simulink model "WF_offshore"  (R2024a)
settings: Solver=VariableStepAuto  StartTime=0  StopTime=1  RelTol=1e-3
values from neighbouring files (symbols this model uses):
  c_c = 0.177e-6    (= 1.77e-07)    [WF_onshore_SSO_GFL.m]    (also in WF_physical_param_offshore_supersynchronous.m = cable_220(i,6)*1e-9; WF_physical_param_onshore_SSO_020625.m = cable_220(i,6)*1e-9; initialize_params_agg.m)
  c_c_eff = c_c*n_cables    [WF_onshore_SSO_GFL.m]    (also in WF_physical_param_offshore_supersynchronous.m; WF_physical_param_onshore_SSO_020625.m; initialize_params_agg.m)
  cvtr = initialize_NR_VSC_GF(cvtr)    [NR_steadystate_VSC_GF.m]    (also in WF_onshore_SSO_GFL.m = setfield(cvtr,'parameters', p_vary.name,p_vary.val(i)); WF_physical_param_offshore_supersynchronous.m = setfield(cvtr,'parameters', p_vary.name,p_vary.val(i)); WF_physical_param_onshore_SSO_020625.m = setfield(cvtr,'parameters', p_vary.name,p_vary.val(i)); impedance_WT_blackbox.m = base_values(cvtr))
  D_C = 10:4:100    [WF_onshore_SSO_GFL.m]    (also in WF_parameter_variation.m = 10:4:150; WF_physical_param.m = 10:4:150; WF_physical_param_offshore_supersynchronous.m = 50; WF_physical_param_onshore_SSO_020625.m = 50)
  enable_pll = 1    [impedance_WT_agg.m]    (also in initialize_WT_agg.m; initialize_WT_default_gfl.m; initialize_WT_default_offshore_super.m)
  f1 = 50    [WF_onshore_SSO_GFL.m]    (also in WF_physical_param_offshore_supersynchronous.m; WF_physical_param_onshore_SSO_020625.m; initialize_params_agg.m)
  i = 1    [WF_physical_param_offshore_supersynchronous.m]    (also in WF_physical_param_onshore_SSO_020625.m)
  L = inv(R)    [participation_factors_VSC_GF.m]
  l_c = 0.386e-3    (= 0.000386)    [WF_onshore_SSO_GFL.m]    (also in WF_physical_param_offshore_supersynchronous.m = cable_220(i,5)*1e-3; WF_physical_param_onshore_SSO_020625.m = cable_220(i,5)*1e-3; initialize_params_agg.m)
  l_c_eff = l_c/n_cables    [WF_onshore_SSO_GFL.m]    (also in WF_physical_param_offshore_supersynchronous.m; WF_physical_param_onshore_SSO_020625.m; initialize_params_agg.m)
  L_comp = sqrt(2)*l_comp*(Z_b_G/(2*pi*f1))    [WF_physical_param.m]    (also in WF_physical_param_offshore_supersynchronous.m = sqrt(2)*((1/(c_c_eff/2*D_C*2*pi*f1))-(l_tf_wf*(Z_b_G)+(l_c_e; WF_physical_param_onshore_SSO_020625.m = sqrt(2)*((1/(c_c_eff/2*D_C*2*pi*f1))-(l_tf_wf*(Z_b_G)+(l_c_e; initialize_params_agg.m)
  l_OH = 0.2    [WF_onshore_SSO_GFL.m]    (also in WF_physical_param_offshore_supersynchronous.m = 0.1; WF_physical_param_onshore_SSO_020625.m = 0.1; initialize_params_agg.m = 0.1)
  l_tf_wf = tf_params(2,2)    [IM_WF_agg.m]    (also in WF_onshore_SSO_GFL.m = 0.05; WF_physical_param_offshore_supersynchronous.m = 0.05; WF_physical_param_onshore_SSO_020625.m = 0.05; initialize_params_agg.m = 0.05)
  l_tf_wt = tf_params(1,2)    [IM_WF_agg.m]    (also in WF_onshore_SSO_GFL.m = 0.0392; WF_physical_param_offshore_supersynchronous.m = 0.0392; WF_physical_param_onshore_SSO_020625.m = 0.0392; initialize_params_agg.m = 0.0392)
  Lg = p_vary(i)*((Z_b_G/(2*pi*f1)))    [WF_onshore_SSO_GFL.m]    (also in WF_physical_param_offshore_supersynchronous.m; WF_physical_param_onshore_SSO_020625.m; initialize_params_agg.m = 0.1*((Z_b_G/(2*pi*f1))))
  Lg1 = Lg    [WF_physical_param_offshore_supersynchronous.m]    (also in WF_physical_param_onshore_SSO_020625.m)
  Lg2 = Lg    [WF_physical_param_offshore_supersynchronous.m]    (also in WF_physical_param_onshore_SSO_020625.m)
  r_c = 27e-3    (= 0.027)    [WF_onshore_SSO_GFL.m]    (also in WF_physical_param_offshore_supersynchronous.m = cable_220(i,4)*1e-3; WF_physical_param_onshore_SSO_020625.m = cable_220(i,4)*1e-3; initialize_params_agg.m)
  r_c_eff = r_c/n_cables    [WF_onshore_SSO_GFL.m]    (also in WF_physical_param_offshore_supersynchronous.m; WF_physical_param_onshore_SSO_020625.m; initialize_params_agg.m)
  r_diss = .1    (= 0.1)    [WF_physical_param_offshore_supersynchronous.m]    (also in WF_physical_param_onshore_SSO_020625.m; calculate_WF.m; initialize_params_agg.m)
  r_OH = 0.02    [WF_onshore_SSO_GFL.m]    (also in WF_physical_param_offshore_supersynchronous.m = 0.01; WF_physical_param_onshore_SSO_020625.m = 0.01; initialize_params_agg.m)
  r_tf_wf = tf_params(2,1)    [IM_WF_agg.m]    (also in WF_onshore_SSO_GFL.m = 0.005; WF_physical_param_offshore_supersynchronous.m = 0.005; WF_physical_param_onshore_SSO_020625.m = 0.005; initialize_params_agg.m = 0.005)
  r_tf_wt = tf_params(1,1)    [IM_WF_agg.m]    (also in WF_onshore_SSO_GFL.m = 0.0056; WF_physical_param_offshore_supersynchronous.m = 0.0056; WF_physical_param_onshore_SSO_020625.m = 0.0056; initialize_params_agg.m = 0.0056)
  Rg = rg*Z_b_G    [WF_onshore_SSO_GFL.m]    (also in WF_physical_param_offshore_supersynchronous.m; WF_physical_param_onshore_SSO_020625.m; initialize_params_agg.m = 0.01*Z_b_G)
  Sb_WF = (3*1)*5e6    (= 15000000)    [WF_onshore_SSO_GFL.m]    (also in WF_physical_param_offshore_supersynchronous.m; WF_physical_param_onshore_SSO_020625.m; impedance_WT_blackbox.m = n_t*Sb_WT; initialize_params_agg.m = 1000000000)
  Sb_WT = 5e6    (= 5000000)    [IM_WF.m]    (also in WF_onshore_SSO_GFL.m; WF_physical_param_offshore_supersynchronous.m; WF_physical_param_onshore_SSO_020625.m; initialize_params_agg.m)
  selector_current_reference = 3    [impedance_WT_agg.m]    (also in initialize_WT_agg.m; initialize_WT_default_gfl.m; initialize_WT_default_offshore_super.m)
  selector_omega_reference = 1    [impedance_WT_agg.m]    (also in initialize_WT_agg.m; initialize_WT_default_gfl.m; initialize_WT_default_offshore_super.m)
  V_coll = 33e3    (= 33000)    [WF_onshore_SSO_GFL.m]    (also in WF_physical_param_offshore_supersynchronous.m; WF_physical_param_onshore_SSO_020625.m; initialize_params_agg.m)
  V_trans = 220e3    (= 220000)    [WF_onshore_SSO_GFL.m]    (also in WF_physical_param_offshore_supersynchronous.m; WF_physical_param_onshore_SSO_020625.m; initialize_params_agg.m)
  Z_b_G = (V_trans/sqrt(3/2))^2/Sb_WF    [WF_onshore_SSO_GFL.m]    (also in WF_physical_param_offshore_supersynchronous.m = (V_b_trans)^2/Sb_WF; WF_physical_param_onshore_SSO_020625.m = (V_b_trans)^2/Sb_WF; initialize_params_agg.m = (V_b_trans)^2/Sb_WF)
undefined symbols (not defined in the file or in its folder): opts, R
libraries: spsSeriesRLCBranchLib x105, simulink_extras x104, simulink x52, spsThreePhaseVIMeasurementLib x42, spsControlledVoltageSourceLib x42, spsGroundLib x41, spsThreePhaseTransformerTwoWindingsLib x14, powerlib_extras x13, spsVariableInductorLib x9, spsIdealSwitchLib x6, spsVariableCapacitorLib x6, spsThreePhaseSeriesRLCBranchLib x4
(part 2 of 13)

== system WF_offshore/WT_MF14 ==
  Control System : Subsystem  mask{Ts_control=cvtr.parameters.T_cont}
      mask prompts: Ts_control "Sample Time"
  Gain1 : Gain  Gain=1/cvtr.pu.Vb
  Gain2 : Gain  Gain=1/cvtr.pu.Ib
  Gain5 : Gain  Gain=cvtr.pu.Vb
  I_conv : ToWorkspace  VariableName=I_conv  SaveFormat=Structure With Time  SampleTime=-1
      settings: MaxDataPoints=1000000
  Inverse Park1 : Subsystem
  Scope2 : Scope  NumInputPorts=2
  Subsystem1 : Subsystem
  Subsystem6 : Subsystem
  Three-Phase Transformer (Two Windings) : spsThreePhaseTransformerTwoWindingsLib/Three-Phase Transformer (Two Windings)  Winding1Connection=Yg  Winding2Connection=Yg  CoreType=Three single-phase transformers  SetSaturation=off  Hysteresis=off  DataFile='hysteresis'  SetInitialFlux=off  Measurements=None  UNITS=pu  NominalPower=[Sb_WF , f1 ]  Winding1=[ cvtr.parameters.Vnr ,r_tf_wt/2 , l_tf_wt/2]  Winding2=[ V_coll , r_tf_wt/2, l_tf_wt/2]  Rm=5000  Lm=0  L0=0.5  Saturation=[ 0,0 ; 0.0024,1.2 ; 1.0,1.52 ]  InitialFluxes=[ 0.8 , -0.8 , 0.7 ]  BreakLoop=off  DiscreteSolver=Trapezoidal iterative  DataType=off  TransfoNumber=1
  Three-Phase V-I Measurement : spsThreePhaseVIMeasurementLib/Three-Phase V-I Measurement  VoltageMeasurement=phase-to-ground  SetLabelV=off  LabelV=Vabc  Vpu=off  VpuLL=off  CurrentMeasurement=yes  SetLabelI=off  LabelI=Iabc  Ipu=off  Pbase=100e6  Vbase=500e3  OutputType=Complex  PhasorSimulation=off  PSBequivalent=0
  Transformations (pu and dq) : Subsystem
  V_conv : ToWorkspace  VariableName=V_conv  SaveFormat=Structure With Time  SampleTime=-1
      settings: MaxDataPoints=1000000
  filter capacitance1 : Subsystem
      settings: PortSchema="{\"entries\":[{\"content\":{\"sides\":[{\"content\":{\"connectorIds\":[\"LConn1\",\"LConn2\",\"LConn3\"]},\"type\":\"ConnectorPlacement.EquallySpacedRectSide\",\"uuid\":\"e81be3d5-6303-4565-8ca3-afc618f21d70\"},{\"content\":{\"connectorIds\":[],\"side\":\"RIGHT\"},\"type\":\"ConnectorPlacement.EquallySpacedRectSide\",\"uuid\":\"458d9030-e614-487d-87de-3e53be7c7da4\"},{\"content\":{\"connectorIds\":[],\"side\":\"TOP\"},\"type\":\"ConnectorPlacement.EquallySpacedRectSide\",\"uuid\":\"a29d66a0-f095-498d-bb9b-96c7f47699d3\"},{\"content\":{\"connectorIds\":[\"Out1\"],\"side\":\"BOTTOM\"},\"type\":\"ConnectorPlacement.EquallySpacedRectSide\",\"uuid\":\"afc68874-c098-43f5-9b37-53a3b484513b\"}]},\"type\":\"ConnectorPlacement.EquallySpacedConnector\",\"uuid\":\"37f495dd-1c12-4bb8-af72-7ef46bbd951c\"}],\"packageUris\":[\"http://schema.mathworks.com/mf0/Connector/R2020b\"],\"version\":\"1.0\"}"
  filter inductance1 : Subsystem
      settings: PortSchema="{\"entries\":[{\"content\":{\"sides\":[{\"content\":{\"connectorIds\":[\"LConn1\",\"LConn2\",\"LConn3\"]},\"type\":\"ConnectorPlacement.EquallySpacedRectSide\",\"uuid\":\"d3d60048-9578-4fa3-8d11-9c8a66a4b1f9\"},{\"content\":{\"connectorIds\":[\"RConn1\",\"RConn2\",\"RConn3\"],\"side\":\"RIGHT\"},\"type\":\"ConnectorPlacement.EquallySpacedRectSide\",\"uuid\":\"184a2c1d-36ab-46d1-99e4-db01aa31ec94\"},{\"content\":{\"connectorIds\":[\"Out1\"],\"side\":\"TOP\"},\"type\":\"ConnectorPlacement.EquallySpacedRectSide\",\"uuid\":\"db651021-9d7f-4124-8d21-ede853163467\"}]},\"type\":\"ConnectorPlacement.EquallySpacedConnector\",\"uuid\":\"723d0964-19fd-4dbe-91e3-e4ea0bb1cca9\"}],\"packageUris\":[\"http://schema.mathworks.com/mf0/Connector/R2020b\"],\"version\":\"1.0\"}"
  a : PMIOPort  Side=Right
  b : PMIOPort  Port=2  Side=Right
  c : PMIOPort  Port=3  Side=Right
  wires:
  Control System/2(thetavsm) -> [Thetavsm]
  Control System/3(vir) -> [vir]
  Control System/1(thetapll) -> [Thetapll]
  Transformations (pu and dq)/2(il) -> Control System/2(il)  "il"
  Transformations (pu and dq)/1(io) -> Control System/1(io)  "io"
  Transformations (pu and dq)/3(p) -> Control System/3(p)  "p"
  Transformations (pu and dq)/4(q) -> Control System/4(q)  "q"
  Transformations (pu and dq)/5(vo_pll) -> Control System/5(vo_pll)  "vo_pll"
  Transformations (pu and dq)/6(vo) -> Control System/6(vo)  "vo"
  [Thetavsm] -> Transformations (pu and dq)/5(Thetavsm)
  [Thetapll] -> Transformations (pu and dq)/6(Thetapll)
  [vir] -> Gain5/1
  Subsystem6/1(x_dq) -> Inverse Park1/1(x_dq)
  Gain5/1 -> Subsystem6/1(x_d+ix_q)
  Three-Phase V-I Measurement/2 -> Gain2/1, [i_abc_grid]  "i_abc_grid"
  Inverse Park1/1(x_abc) -> Subsystem1/1(v_abc)
  Three-Phase V-I Measurement/1 -> Gain1/1, [v_abc_grid]  "v_abc_grid"
  [Thetavsm] -> Inverse Park1/2(delta)
  filter capacitance1/1(v_abc) -> [v_abc_filt]  "v_abc_filt"
  filter inductance1/1(i_abc) -> [i_abc_filt]  "i_abc_filt"
  [v_abc_grid] -> Transformations (pu and dq)/3(v_abc_grid)
  [v_abc_filt] -> Transformations (pu and dq)/4(v_abc_filt)
  [i_abc_filt] -> Transformations (pu and dq)/2(i_abc_filt)
  [i_abc_grid] -> Transformations (pu and dq)/1(i_abc_grid)
  Gain1/1 -> Scope2/1, V_conv/1
  Gain2/1 -> Scope2/2, I_conv/1
  connections:
  filter inductance1/RConn3 -- filter capacitance1/LConn3 -- Three-Phase V-I Measurement/LConn3
  filter inductance1/RConn1 -- filter capacitance1/LConn1 -- Three-Phase V-I Measurement/LConn1
  filter inductance1/RConn2 -- filter capacitance1/LConn2 -- Three-Phase V-I Measurement/LConn2
  Subsystem1/RConn1 -- filter inductance1/LConn1
  Subsystem1/RConn2 -- filter inductance1/LConn2
  Subsystem1/RConn3 -- filter inductance1/LConn3
  Three-Phase Transformer (Two Windings)/RConn1 -- a/RConn1
  Three-Phase Transformer (Two Windings)/RConn2 -- b/RConn1
  Three-Phase Transformer (Two Windings)/RConn3 -- c/RConn1
  Three-Phase Transformer (Two Windings)/LConn1 -- Three-Phase V-I Measurement/RConn1
  Three-Phase Transformer (Two Windings)/LConn2 -- Three-Phase V-I Measurement/RConn2
  Three-Phase Transformer (Two Windings)/LConn3 -- Three-Phase V-I Measurement/RConn3

== system WF_offshore/WT_MF2 ==
  Control System : Subsystem  mask{Ts_control=cvtr.parameters.T_cont}
      mask prompts: Ts_control "Sample Time"
  Gain5 : Gain  Gain=cvtr.pu.Vb
  Inverse Park1 : Subsystem
  Subsystem1 : Subsystem
  Subsystem6 : Subsystem
  Three-Phase Transformer (Two Windings) : spsThreePhaseTransformerTwoWindingsLib/Three-Phase Transformer (Two Windings)  Winding1Connection=Yg  Winding2Connection=Yg  CoreType=Three single-phase transformers  SetSaturation=off  Hysteresis=off  DataFile='hysteresis'  SetInitialFlux=off  Measurements=None  UNITS=pu  NominalPower=[Sb_WT, f1 ]  Winding1=[ cvtr.parameters.Vnr ,r_tf_wt/2 , l_tf_wt/2]  Winding2=[ V_coll , r_tf_wt/2, l_tf_wt/2]  Rm=5000  Lm=0  L0=0.5  Saturation=[ 0,0 ; 0.0024,1.2 ; 1.0,1.52 ]  InitialFluxes=[ 0.8 , -0.8 , 0.7 ]  BreakLoop=off  DiscreteSolver=Trapezoidal iterative  DataType=off  TransfoNumber=1
  Three-Phase V-I Measurement : spsThreePhaseVIMeasurementLib/Three-Phase V-I Measurement  VoltageMeasurement=phase-to-ground  SetLabelV=off  LabelV=Vabc  Vpu=off  VpuLL=off  CurrentMeasurement=yes  SetLabelI=off  LabelI=Iabc  Ipu=off  Pbase=100e6  Vbase=500e3  OutputType=Complex  PhasorSimulation=off  PSBequivalent=0
  Transformations (pu and dq) : Subsystem
  filter capacitance1 : Subsystem
      settings: PortSchema="{\"entries\":[{\"content\":{\"sides\":[{\"content\":{\"connectorIds\":[\"LConn1\",\"LConn2\",\"LConn3\"]},\"type\":\"ConnectorPlacement.EquallySpacedRectSide\",\"uuid\":\"e81be3d5-6303-4565-8ca3-afc618f21d70\"},{\"content\":{\"connectorIds\":[],\"side\":\"RIGHT\"},\"type\":\"ConnectorPlacement.EquallySpacedRectSide\",\"uuid\":\"458d9030-e614-487d-87de-3e53be7c7da4\"},{\"content\":{\"connectorIds\":[],\"side\":\"TOP\"},\"type\":\"ConnectorPlacement.EquallySpacedRectSide\",\"uuid\":\"a29d66a0-f095-498d-bb9b-96c7f47699d3\"},{\"content\":{\"connectorIds\":[\"Out1\"],\"side\":\"BOTTOM\"},\"type\":\"ConnectorPlacement.EquallySpacedRectSide\",\"uuid\":\"afc68874-c098-43f5-9b37-53a3b484513b\"}]},\"type\":\"ConnectorPlacement.EquallySpacedConnector\",\"uuid\":\"37f495dd-1c12-4bb8-af72-7ef46bbd951c\"}],\"packageUris\":[\"http://schema.mathworks.com/mf0/Connector/R2020b\"],\"version\":\"1.0\"}"
  filter inductance1 : Subsystem
      settings: PortSchema="{\"entries\":[{\"content\":{\"sides\":[{\"content\":{\"connectorIds\":[\"LConn1\",\"LConn2\",\"LConn3\"]},\"type\":\"ConnectorPlacement.EquallySpacedRectSide\",\"uuid\":\"d3d60048-9578-4fa3-8d11-9c8a66a4b1f9\"},{\"content\":{\"connectorIds\":[\"RConn1\",\"RConn2\",\"RConn3\"],\"side\":\"RIGHT\"},\"type\":\"ConnectorPlacement.EquallySpacedRectSide\",\"uuid\":\"184a2c1d-36ab-46d1-99e4-db01aa31ec94\"},{\"content\":{\"connectorIds\":[\"Out1\"],\"side\":\"TOP\"},\"type\":\"ConnectorPlacement.EquallySpacedRectSide\",\"uuid\":\"db651021-9d7f-4124-8d21-ede853163467\"}]},\"type\":\"ConnectorPlacement.EquallySpacedConnector\",\"uuid\":\"723d0964-19fd-4dbe-91e3-e4ea0bb1cca9\"}],\"packageUris\":[\"http://schema.mathworks.com/mf0/Connector/R2020b\"],\"version\":\"1.0\"}"
  a : PMIOPort  Side=Right
  b : PMIOPort  Port=2  Side=Right
  c : PMIOPort  Port=3  Side=Right
  wires:
  [i_abc_grid] -> Transformations (pu and dq)/1(i_abc_grid)
  [i_abc_filt] -> Transformations (pu and dq)/2(i_abc_filt)
  [v_abc_filt] -> Transformations (pu and dq)/4(v_abc_filt)
  [v_abc_grid] -> Transformations (pu and dq)/3(v_abc_grid)
  filter inductance1/1(i_abc) -> [i_abc_filt]  "i_abc_filt"
  filter capacitance1/1(v_abc) -> [v_abc_filt]  "v_abc_filt"
  [Thetavsm] -> Inverse Park1/2(delta)
  Three-Phase V-I Measurement/1 -> [v_abc_grid]  "v_abc_grid"
  Inverse Park1/1(x_abc) -> Subsystem1/1(v_abc)
  Three-Phase V-I Measurement/2 -> [i_abc_grid]  "i_abc_grid"
  Gain5/1 -> Subsystem6/1(x_d+ix_q)
  Subsystem6/1(x_dq) -> Inverse Park1/1(x_dq)
  [vir] -> Gain5/1
  [Thetapll] -> Transformations (pu and dq)/6(Thetapll)
  [Thetavsm] -> Transformations (pu and dq)/5(Thetavsm)
  Transformations (pu and dq)/6(vo) -> Control System/6(vo)  "vo"
  Transformations (pu and dq)/5(vo_pll) -> Control System/5(vo_pll)  "vo_pll"
  Transformations (pu and dq)/4(q) -> Control System/4(q)  "q"
  Transformations (pu and dq)/3(p) -> Control System/3(p)  "p"
  Transformations (pu and dq)/1(io) -> Control System/1(io)  "io"
  Transformations (pu and dq)/2(il) -> Control System/2(il)  "il"
  Control System/1(thetapll) -> [Thetapll]
  Control System/3(vir) -> [vir]
  Control System/2(thetavsm) -> [Thetavsm]
  connections:
  Three-Phase Transformer (Two Windings)/LConn3 -- Three-Phase V-I Measurement/RConn3
  Three-Phase Transformer (Two Windings)/LConn2 -- Three-Phase V-I Measurement/RConn2
  Three-Phase Transformer (Two Windings)/LConn1 -- Three-Phase V-I Measurement/RConn1
  Three-Phase Transformer (Two Windings)/RConn3 -- c/RConn1
  Three-Phase Transformer (Two Windings)/RConn2 -- b/RConn1
  Three-Phase Transformer (Two Windings)/RConn1 -- a/RConn1
  Subsystem1/RConn3 -- filter inductance1/LConn3
  Subsystem1/RConn2 -- filter inductance1/LConn2
  Subsystem1/RConn1 -- filter inductance1/LConn1
  Three-Phase V-I Measurement/LConn2 -- filter capacitance1/LConn2 -- filter inductance1/RConn2
  Three-Phase V-I Measurement/LConn1 -- filter capacitance1/LConn1 -- filter inductance1/RConn1
  Three-Phase V-I Measurement/LConn3 -- filter capacitance1/LConn3 -- filter inductance1/RConn3

== system WF_offshore/WT_MF3 ==
  Control System : Subsystem  mask{Ts_control=cvtr.parameters.T_cont}
      mask prompts: Ts_control "Sample Time"
  Gain5 : Gain  Gain=cvtr.pu.Vb
  Inverse Park1 : Subsystem
  Subsystem1 : Subsystem
  Subsystem6 : Subsystem
  Three-Phase Transformer (Two Windings) : spsThreePhaseTransformerTwoWindingsLib/Three-Phase Transformer (Two Windings)  Winding1Connection=Yg  Winding2Connection=Yg  CoreType=Three single-phase transformers  SetSaturation=off  Hysteresis=off  DataFile='hysteresis'  SetInitialFlux=off  Measurements=None  UNITS=pu  NominalPower=[Sb_WT, f1 ]  Winding1=[ cvtr.parameters.Vnr ,r_tf_wt/2 , l_tf_wt/2]  Winding2=[ V_coll , r_tf_wt/2, l_tf_wt/2]  Rm=5000  Lm=0  L0=0.5  Saturation=[ 0,0 ; 0.0024,1.2 ; 1.0,1.52 ]  InitialFluxes=[ 0.8 , -0.8 , 0.7 ]  BreakLoop=off  DiscreteSolver=Trapezoidal iterative  DataType=off  TransfoNumber=1
  Three-Phase V-I Measurement : spsThreePhaseVIMeasurementLib/Three-Phase V-I Measurement  VoltageMeasurement=phase-to-ground  SetLabelV=off  LabelV=Vabc  Vpu=off  VpuLL=off  CurrentMeasurement=yes  SetLabelI=off  LabelI=Iabc  Ipu=off  Pbase=100e6  Vbase=500e3  OutputType=Complex  PhasorSimulation=off  PSBequivalent=0
  Transformations (pu and dq) : Subsystem
  filter capacitance1 : Subsystem
      settings: PortSchema="{\"entries\":[{\"content\":{\"sides\":[{\"content\":{\"connectorIds\":[\"LConn1\",\"LConn2\",\"LConn3\"]},\"type\":\"ConnectorPlacement.EquallySpacedRectSide\",\"uuid\":\"e81be3d5-6303-4565-8ca3-afc618f21d70\"},{\"content\":{\"connectorIds\":[],\"side\":\"RIGHT\"},\"type\":\"ConnectorPlacement.EquallySpacedRectSide\",\"uuid\":\"458d9030-e614-487d-87de-3e53be7c7da4\"},{\"content\":{\"connectorIds\":[],\"side\":\"TOP\"},\"type\":\"ConnectorPlacement.EquallySpacedRectSide\",\"uuid\":\"a29d66a0-f095-498d-bb9b-96c7f47699d3\"},{\"content\":{\"connectorIds\":[\"Out1\"],\"side\":\"BOTTOM\"},\"type\":\"ConnectorPlacement.EquallySpacedRectSide\",\"uuid\":\"afc68874-c098-43f5-9b37-53a3b484513b\"}]},\"type\":\"ConnectorPlacement.EquallySpacedConnector\",\"uuid\":\"37f495dd-1c12-4bb8-af72-7ef46bbd951c\"}],\"packageUris\":[\"http://schema.mathworks.com/mf0/Connector/R2020b\"],\"version\":\"1.0\"}"
  filter inductance1 : Subsystem
      settings: PortSchema="{\"entries\":[{\"content\":{\"sides\":[{\"content\":{\"connectorIds\":[\"LConn1\",\"LConn2\",\"LConn3\"]},\"type\":\"ConnectorPlacement.EquallySpacedRectSide\",\"uuid\":\"d3d60048-9578-4fa3-8d11-9c8a66a4b1f9\"},{\"content\":{\"connectorIds\":[\"RConn1\",\"RConn2\",\"RConn3\"],\"side\":\"RIGHT\"},\"type\":\"ConnectorPlacement.EquallySpacedRectSide\",\"uuid\":\"184a2c1d-36ab-46d1-99e4-db01aa31ec94\"},{\"content\":{\"connectorIds\":[\"Out1\"],\"side\":\"TOP\"},\"type\":\"ConnectorPlacement.EquallySpacedRectSide\",\"uuid\":\"db651021-9d7f-4124-8d21-ede853163467\"}]},\"type\":\"ConnectorPlacement.EquallySpacedConnector\",\"uuid\":\"723d0964-19fd-4dbe-91e3-e4ea0bb1cca9\"}],\"packageUris\":[\"http://schema.mathworks.com/mf0/Connector/R2020b\"],\"version\":\"1.0\"}"
  a : PMIOPort  Side=Right
  b : PMIOPort  Port=2  Side=Right
  c : PMIOPort  Port=3  Side=Right
  wires:
  Control System/2(thetavsm) -> [Thetavsm]
  Control System/3(vir) -> [vir]
  Control System/1(thetapll) -> [Thetapll]
  Transformations (pu and dq)/2(il) -> Control System/2(il)  "il"
  Transformations (pu and dq)/1(io) -> Control System/1(io)  "io"
  Transformations (pu and dq)/3(p) -> Control System/3(p)  "p"
  Transformations (pu and dq)/4(q) -> Control System/4(q)  "q"
  Transformations (pu and dq)/5(vo_pll) -> Control System/5(vo_pll)  "vo_pll"
  Transformations (pu and dq)/6(vo) -> Control System/6(vo)  "vo"
  [Thetavsm] -> Transformations (pu and dq)/5(Thetavsm)
  [Thetapll] -> Transformations (pu and dq)/6(Thetapll)
  [vir] -> Gain5/1
  Subsystem6/1(x_dq) -> Inverse Park1/1(x_dq)
  Gain5/1 -> Subsystem6/1(x_d+ix_q)
  Three-Phase V-I Measurement/2 -> [i_abc_grid]  "i_abc_grid"
  Inverse Park1/1(x_abc) -> Subsystem1/1(v_abc)
  Three-Phase V-I Measurement/1 -> [v_abc_grid]  "v_abc_grid"
  [Thetavsm] -> Inverse Park1/2(delta)
  filter capacitance1/1(v_abc) -> [v_abc_filt]  "v_abc_filt"
  filter inductance1/1(i_abc) -> [i_abc_filt]  "i_abc_filt"
  [v_abc_grid] -> Transformations (pu and dq)/3(v_abc_grid)
  [v_abc_filt] -> Transformations (pu and dq)/4(v_abc_filt)
  [i_abc_filt] -> Transformations (pu and dq)/2(i_abc_filt)
  [i_abc_grid] -> Transformations (pu and dq)/1(i_abc_grid)
  connections:
  filter inductance1/RConn3 -- filter capacitance1/LConn3 -- Three-Phase V-I Measurement/LConn3
  filter inductance1/RConn1 -- filter capacitance1/LConn1 -- Three-Phase V-I Measurement/LConn1
  filter inductance1/RConn2 -- filter capacitance1/LConn2 -- Three-Phase V-I Measurement/LConn2
  Subsystem1/RConn1 -- filter inductance1/LConn1
  Subsystem1/RConn2 -- filter inductance1/LConn2
  Subsystem1/RConn3 -- filter inductance1/LConn3
  Three-Phase Transformer (Two Windings)/RConn1 -- a/RConn1
  Three-Phase Transformer (Two Windings)/RConn2 -- b/RConn1
  Three-Phase Transformer (Two Windings)/RConn3 -- c/RConn1
  Three-Phase Transformer (Two Windings)/LConn1 -- Three-Phase V-I Measurement/RConn1
  Three-Phase Transformer (Two Windings)/LConn2 -- Three-Phase V-I Measurement/RConn2
  Three-Phase Transformer (Two Windings)/LConn3 -- Three-Phase V-I Measurement/RConn3

== system WF_offshore/WT_MF4 ==
  Control System : Subsystem  mask{Ts_control=cvtr.parameters.T_cont}
      mask prompts: Ts_control "Sample Time"
  Gain5 : Gain  Gain=cvtr.pu.Vb
  Inverse Park1 : Subsystem
  Subsystem1 : Subsystem
  Subsystem6 : Subsystem
  Three-Phase Transformer (Two Windings) : spsThreePhaseTransformerTwoWindingsLib/Three-Phase Transformer (Two Windings)  Winding1Connection=Yg  Winding2Connection=Yg  CoreType=Three single-phase transformers  SetSaturation=off  Hysteresis=off  DataFile='hysteresis'  SetInitialFlux=off  Measurements=None  UNITS=pu  NominalPower=[Sb_WT, f1 ]  Winding1=[ cvtr.parameters.Vnr ,r_tf_wt/2 , l_tf_wt/2]  Winding2=[ V_coll , r_tf_wt/2, l_tf_wt/2]  Rm=5000  Lm=0  L0=0.5  Saturation=[ 0,0 ; 0.0024,1.2 ; 1.0,1.52 ]  InitialFluxes=[ 0.8 , -0.8 , 0.7 ]  BreakLoop=off  DiscreteSolver=Trapezoidal iterative  DataType=off  TransfoNumber=1
  Three-Phase V-I Measurement : spsThreePhaseVIMeasurementLib/Three-Phase V-I Measurement  VoltageMeasurement=phase-to-ground  SetLabelV=off  LabelV=Vabc  Vpu=off  VpuLL=off  CurrentMeasurement=yes  SetLabelI=off  LabelI=Iabc  Ipu=off  Pbase=100e6  Vbase=500e3  OutputType=Complex  PhasorSimulation=off  PSBequivalent=0
  Transformations (pu and dq) : Subsystem
  filter capacitance1 : Subsystem
      settings: PortSchema="{\"entries\":[{\"content\":{\"sides\":[{\"content\":{\"connectorIds\":[\"LConn1\",\"LConn2\",\"LConn3\"]},\"type\":\"ConnectorPlacement.EquallySpacedRectSide\",\"uuid\":\"e81be3d5-6303-4565-8ca3-afc618f21d70\"},{\"content\":{\"connectorIds\":[],\"side\":\"RIGHT\"},\"type\":\"ConnectorPlacement.EquallySpacedRectSide\",\"uuid\":\"458d9030-e614-487d-87de-3e53be7c7da4\"},{\"content\":{\"connectorIds\":[],\"side\":\"TOP\"},\"type\":\"ConnectorPlacement.EquallySpacedRectSide\",\"uuid\":\"a29d66a0-f095-498d-bb9b-96c7f47699d3\"},{\"content\":{\"connectorIds\":[\"Out1\"],\"side\":\"BOTTOM\"},\"type\":\"ConnectorPlacement.EquallySpacedRectSide\",\"uuid\":\"afc68874-c098-43f5-9b37-53a3b484513b\"}]},\"type\":\"ConnectorPlacement.EquallySpacedConnector\",\"uuid\":\"37f495dd-1c12-4bb8-af72-7ef46bbd951c\"}],\"packageUris\":[\"http://schema.mathworks.com/mf0/Connector/R2020b\"],\"version\":\"1.0\"}"
  filter inductance1 : Subsystem
      settings: PortSchema="{\"entries\":[{\"content\":{\"sides\":[{\"content\":{\"connectorIds\":[\"LConn1\",\"LConn2\",\"LConn3\"]},\"type\":\"ConnectorPlacement.EquallySpacedRectSide\",\"uuid\":\"d3d60048-9578-4fa3-8d11-9c8a66a4b1f9\"},{\"content\":{\"connectorIds\":[\"RConn1\",\"RConn2\",\"RConn3\"],\"side\":\"RIGHT\"},\"type\":\"ConnectorPlacement.EquallySpacedRectSide\",\"uuid\":\"184a2c1d-36ab-46d1-99e4-db01aa31ec94\"},{\"content\":{\"connectorIds\":[\"Out1\"],\"side\":\"TOP\"},\"type\":\"ConnectorPlacement.EquallySpacedRectSide\",\"uuid\":\"db651021-9d7f-4124-8d21-ede853163467\"}]},\"type\":\"ConnectorPlacement.EquallySpacedConnector\",\"uuid\":\"723d0964-19fd-4dbe-91e3-e4ea0bb1cca9\"}],\"packageUris\":[\"http://schema.mathworks.com/mf0/Connector/R2020b\"],\"version\":\"1.0\"}"
  a : PMIOPort  Side=Right
  b : PMIOPort  Port=2  Side=Right
  c : PMIOPort  Port=3  Side=Right
  wires:
  [i_abc_grid] -> Transformations (pu and dq)/1(i_abc_grid)
  [i_abc_filt] -> Transformations (pu and dq)/2(i_abc_filt)
  [v_abc_filt] -> Transformations (pu and dq)/4(v_abc_filt)
  [v_abc_grid] -> Transformations (pu and dq)/3(v_abc_grid)
  filter inductance1/1(i_abc) -> [i_abc_filt]  "i_abc_filt"
  filter capacitance1/1(v_abc) -> [v_abc_filt]  "v_abc_filt"
  [Thetavsm] -> Inverse Park1/2(delta)
  Three-Phase V-I Measurement/1 -> [v_abc_grid]  "v_abc_grid"
  Inverse Park1/1(x_abc) -> Subsystem1/1(v_abc)
  Three-Phase V-I Measurement/2 -> [i_abc_grid]  "i_abc_grid"
  Gain5/1 -> Subsystem6/1(x_d+ix_q)
  Subsystem6/1(x_dq) -> Inverse Park1/1(x_dq)
  [vir] -> Gain5/1
  [Thetapll] -> Transformations (pu and dq)/6(Thetapll)
  [Thetavsm] -> Transformations (pu and dq)/5(Thetavsm)
  Transformations (pu and dq)/6(vo) -> Control System/6(vo)  "vo"
  Transformations (pu and dq)/5(vo_pll) -> Control System/5(vo_pll)  "vo_pll"
  Transformations (pu and dq)/4(q) -> Control System/4(q)  "q"
  Transformations (pu and dq)/3(p) -> Control System/3(p)  "p"
  Transformations (pu and dq)/1(io) -> Control System/1(io)  "io"
  Transformations (pu and dq)/2(il) -> Control System/2(il)  "il"
  Control System/1(thetapll) -> [Thetapll]
  Control System/3(vir) -> [vir]
  Control System/2(thetavsm) -> [Thetavsm]
  connections:
  Three-Phase Transformer (Two Windings)/LConn3 -- Three-Phase V-I Measurement/RConn3
  Three-Phase Transformer (Two Windings)/LConn2 -- Three-Phase V-I Measurement/RConn2
  Three-Phase Transformer (Two Windings)/LConn1 -- Three-Phase V-I Measurement/RConn1
  Three-Phase Transformer (Two Windings)/RConn3 -- c/RConn1
  Three-Phase Transformer (Two Windings)/RConn2 -- b/RConn1
  Three-Phase Transformer (Two Windings)/RConn1 -- a/RConn1
  Subsystem1/RConn3 -- filter inductance1/LConn3
  Subsystem1/RConn2 -- filter inductance1/LConn2
  Subsystem1/RConn1 -- filter inductance1/LConn1
  Three-Phase V-I Measurement/LConn2 -- filter capacitance1/LConn2 -- filter inductance1/RConn2
  Three-Phase V-I Measurement/LConn1 -- filter capacitance1/LConn1 -- filter inductance1/RConn1
  Three-Phase V-I Measurement/LConn3 -- filter capacitance1/LConn3 -- filter inductance1/RConn3

== system WF_offshore/WT_MF5 ==
  Control System : Subsystem  mask{Ts_control=cvtr.parameters.T_cont}
      mask prompts: Ts_control "Sample Time"
  Gain5 : Gain  Gain=cvtr.pu.Vb
  Inverse Park1 : Subsystem
  Subsystem1 : Subsystem
  Subsystem6 : Subsystem
  Three-Phase Transformer (Two Windings) : spsThreePhaseTransformerTwoWindingsLib/Three-Phase Transformer (Two Windings)  Winding1Connection=Yg  Winding2Connection=Yg  CoreType=Three single-phase transformers  SetSaturation=off  Hysteresis=off  DataFile='hysteresis'  SetInitialFlux=off  Measurements=None  UNITS=pu  NominalPower=[Sb_WT, f1 ]  Winding1=[ cvtr.parameters.Vnr ,r_tf_wt/2 , l_tf_wt/2]  Winding2=[ V_coll , r_tf_wt/2, l_tf_wt/2]  Rm=5000  Lm=0  L0=0.5  Saturation=[ 0,0 ; 0.0024,1.2 ; 1.0,1.52 ]  InitialFluxes=[ 0.8 , -0.8 , 0.7 ]  BreakLoop=off  DiscreteSolver=Trapezoidal iterative  DataType=off  TransfoNumber=1
  Three-Phase V-I Measurement : spsThreePhaseVIMeasurementLib/Three-Phase V-I Measurement  VoltageMeasurement=phase-to-ground  SetLabelV=off  LabelV=Vabc  Vpu=off  VpuLL=off  CurrentMeasurement=yes  SetLabelI=off  LabelI=Iabc  Ipu=off  Pbase=100e6  Vbase=500e3  OutputType=Complex  PhasorSimulation=off  PSBequivalent=0
  Transformations (pu and dq) : Subsystem
  filter capacitance1 : Subsystem
      settings: PortSchema="{\"entries\":[{\"content\":{\"sides\":[{\"content\":{\"connectorIds\":[\"LConn1\",\"LConn2\",\"LConn3\"]},\"type\":\"ConnectorPlacement.EquallySpacedRectSide\",\"uuid\":\"e81be3d5-6303-4565-8ca3-afc618f21d70\"},{\"content\":{\"connectorIds\":[],\"side\":\"RIGHT\"},\"type\":\"ConnectorPlacement.EquallySpacedRectSide\",\"uuid\":\"458d9030-e614-487d-87de-3e53be7c7da4\"},{\"content\":{\"connectorIds\":[],\"side\":\"TOP\"},\"type\":\"ConnectorPlacement.EquallySpacedRectSide\",\"uuid\":\"a29d66a0-f095-498d-bb9b-96c7f47699d3\"},{\"content\":{\"connectorIds\":[\"Out1\"],\"side\":\"BOTTOM\"},\"type\":\"ConnectorPlacement.EquallySpacedRectSide\",\"uuid\":\"afc68874-c098-43f5-9b37-53a3b484513b\"}]},\"type\":\"ConnectorPlacement.EquallySpacedConnector\",\"uuid\":\"37f495dd-1c12-4bb8-af72-7ef46bbd951c\"}],\"packageUris\":[\"http://schema.mathworks.com/mf0/Connector/R2020b\"],\"version\":\"1.0\"}"
  filter inductance1 : Subsystem
      settings: PortSchema="{\"entries\":[{\"content\":{\"sides\":[{\"content\":{\"connectorIds\":[\"LConn1\",\"LConn2\",\"LConn3\"]},\"type\":\"ConnectorPlacement.EquallySpacedRectSide\",\"uuid\":\"d3d60048-9578-4fa3-8d11-9c8a66a4b1f9\"},{\"content\":{\"connectorIds\":[\"RConn1\",\"RConn2\",\"RConn3\"],\"side\":\"RIGHT\"},\"type\":\"ConnectorPlacement.EquallySpacedRectSide\",\"uuid\":\"184a2c1d-36ab-46d1-99e4-db01aa31ec94\"},{\"content\":{\"connectorIds\":[\"Out1\"],\"side\":\"TOP\"},\"type\":\"ConnectorPlacement.EquallySpacedRectSide\",\"uuid\":\"db651021-9d7f-4124-8d21-ede853163467\"}]},\"type\":\"ConnectorPlacement.EquallySpacedConnector\",\"uuid\":\"723d0964-19fd-4dbe-91e3-e4ea0bb1cca9\"}],\"packageUris\":[\"http://schema.mathworks.com/mf0/Connector/R2020b\"],\"version\":\"1.0\"}"
  a : PMIOPort  Side=Right
  b : PMIOPort  Port=2  Side=Right
  c : PMIOPort  Port=3  Side=Right
  wires:
  Control System/2(thetavsm) -> [Thetavsm]
  Control System/3(vir) -> [vir]
  Control System/1(thetapll) -> [Thetapll]
  Transformations (pu and dq)/2(il) -> Control System/2(il)  "il"
  Transformations (pu and dq)/1(io) -> Control System/1(io)  "io"
  Transformations (pu and dq)/3(p) -> Control System/3(p)  "p"
  Transformations (pu and dq)/4(q) -> Control System/4(q)  "q"
  Transformations (pu and dq)/5(vo_pll) -> Control System/5(vo_pll)  "vo_pll"
  Transformations (pu and dq)/6(vo) -> Control System/6(vo)  "vo"
  [Thetavsm] -> Transformations (pu and dq)/5(Thetavsm)
  [Thetapll] -> Transformations (pu and dq)/6(Thetapll)
  [vir] -> Gain5/1
  Subsystem6/1(x_dq) -> Inverse Park1/1(x_dq)
  Gain5/1 -> Subsystem6/1(x_d+ix_q)
  Three-Phase V-I Measurement/2 -> [i_abc_grid]  "i_abc_grid"
  Inverse Park1/1(x_abc) -> Subsystem1/1(v_abc)
  Three-Phase V-I Measurement/1 -> [v_abc_grid]  "v_abc_grid"
  [Thetavsm] -> Inverse Park1/2(delta)
  filter capacitance1/1(v_abc) -> [v_abc_filt]  "v_abc_filt"
  filter inductance1/1(i_abc) -> [i_abc_filt]  "i_abc_filt"
  [v_abc_grid] -> Transformations (pu and dq)/3(v_abc_grid)
  [v_abc_filt] -> Transformations (pu and dq)/4(v_abc_filt)
  [i_abc_filt] -> Transformations (pu and dq)/2(i_abc_filt)
  [i_abc_grid] -> Transformations (pu and dq)/1(i_abc_grid)
  connections:
  filter inductance1/RConn3 -- filter capacitance1/LConn3 -- Three-Phase V-I Measurement/LConn3
  filter inductance1/RConn1 -- filter capacitance1/LConn1 -- Three-Phase V-I Measurement/LConn1
  filter inductance1/RConn2 -- filter capacitance1/LConn2 -- Three-Phase V-I Measurement/LConn2
  Subsystem1/RConn1 -- filter inductance1/LConn1
  Subsystem1/RConn2 -- filter inductance1/LConn2
  Subsystem1/RConn3 -- filter inductance1/LConn3
  Three-Phase Transformer (Two Windings)/RConn1 -- a/RConn1
  Three-Phase Transformer (Two Windings)/RConn2 -- b/RConn1
  Three-Phase Transformer (Two Windings)/RConn3 -- c/RConn1
  Three-Phase Transformer (Two Windings)/LConn1 -- Three-Phase V-I Measurement/RConn1
  Three-Phase Transformer (Two Windings)/LConn2 -- Three-Phase V-I Measurement/RConn2
  Three-Phase Transformer (Two Windings)/LConn3 -- Three-Phase V-I Measurement/RConn3

== system WF_offshore/WT_MF6 ==
  Control System : Subsystem  mask{Ts_control=cvtr.parameters.T_cont}
      mask prompts: Ts_control "Sample Time"
  Gain5 : Gain  Gain=cvtr.pu.Vb
  Inverse Park1 : Subsystem
  Subsystem1 : Subsystem
  Subsystem6 : Subsystem
  Three-Phase Transformer (Two Windings) : spsThreePhaseTransformerTwoWindingsLib/Three-Phase Transformer (Two Windings)  Winding1Connection=Yg  Winding2Connection=Yg  CoreType=Three single-phase transformers  SetSaturation=off  Hysteresis=off  DataFile='hysteresis'  SetInitialFlux=off  Measurements=None  UNITS=pu  NominalPower=[Sb_WT, f1 ]  Winding1=[ cvtr.parameters.Vnr ,r_tf_wt/2 , l_tf_wt/2]  Winding2=[ V_coll , r_tf_wt/2, l_tf_wt/2]  Rm=5000  Lm=0  L0=0.5  Saturation=[ 0,0 ; 0.0024,1.2 ; 1.0,1.52 ]  InitialFluxes=[ 0.8 , -0.8 , 0.7 ]  BreakLoop=off  DiscreteSolver=Trapezoidal iterative  DataType=off  TransfoNumber=1
  Three-Phase V-I Measurement : spsThreePhaseVIMeasurementLib/Three-Phase V-I Measurement  VoltageMeasurement=phase-to-ground  SetLabelV=off  LabelV=Vabc  Vpu=off  VpuLL=off  CurrentMeasurement=yes  SetLabelI=off  LabelI=Iabc  Ipu=off  Pbase=100e6  Vbase=500e3  OutputType=Complex  PhasorSimulation=off  PSBequivalent=0
  Transformations (pu and dq) : Subsystem
  filter capacitance1 : Subsystem
      settings: PortSchema="{\"entries\":[{\"content\":{\"sides\":[{\"content\":{\"connectorIds\":[\"LConn1\",\"LConn2\",\"LConn3\"]},\"type\":\"ConnectorPlacement.EquallySpacedRectSide\",\"uuid\":\"e81be3d5-6303-4565-8ca3-afc618f21d70\"},{\"content\":{\"connectorIds\":[],\"side\":\"RIGHT\"},\"type\":\"ConnectorPlacement.EquallySpacedRectSide\",\"uuid\":\"458d9030-e614-487d-87de-3e53be7c7da4\"},{\"content\":{\"connectorIds\":[],\"side\":\"TOP\"},\"type\":\"ConnectorPlacement.EquallySpacedRectSide\",\"uuid\":\"a29d66a0-f095-498d-bb9b-96c7f47699d3\"},{\"content\":{\"connectorIds\":[\"Out1\"],\"side\":\"BOTTOM\"},\"type\":\"ConnectorPlacement.EquallySpacedRectSide\",\"uuid\":\"afc68874-c098-43f5-9b37-53a3b484513b\"}]},\"type\":\"ConnectorPlacement.EquallySpacedConnector\",\"uuid\":\"37f495dd-1c12-4bb8-af72-7ef46bbd951c\"}],\"packageUris\":[\"http://schema.mathworks.com/mf0/Connector/R2020b\"],\"version\":\"1.0\"}"
  filter inductance1 : Subsystem
      settings: PortSchema="{\"entries\":[{\"content\":{\"sides\":[{\"content\":{\"connectorIds\":[\"LConn1\",\"LConn2\",\"LConn3\"]},\"type\":\"ConnectorPlacement.EquallySpacedRectSide\",\"uuid\":\"d3d60048-9578-4fa3-8d11-9c8a66a4b1f9\"},{\"content\":{\"connectorIds\":[\"RConn1\",\"RConn2\",\"RConn3\"],\"side\":\"RIGHT\"},\"type\":\"ConnectorPlacement.EquallySpacedRectSide\",\"uuid\":\"184a2c1d-36ab-46d1-99e4-db01aa31ec94\"},{\"content\":{\"connectorIds\":[\"Out1\"],\"side\":\"TOP\"},\"type\":\"ConnectorPlacement.EquallySpacedRectSide\",\"uuid\":\"db651021-9d7f-4124-8d21-ede853163467\"}]},\"type\":\"ConnectorPlacement.EquallySpacedConnector\",\"uuid\":\"723d0964-19fd-4dbe-91e3-e4ea0bb1cca9\"}],\"packageUris\":[\"http://schema.mathworks.com/mf0/Connector/R2020b\"],\"version\":\"1.0\"}"
  a : PMIOPort  Side=Right
  b : PMIOPort  Port=2  Side=Right
  c : PMIOPort  Port=3  Side=Right
  wires:
  [i_abc_grid] -> Transformations (pu and dq)/1(i_abc_grid)
  [i_abc_filt] -> Transformations (pu and dq)/2(i_abc_filt)
  [v_abc_filt] -> Transformations (pu and dq)/4(v_abc_filt)
  [v_abc_grid] -> Transformations (pu and dq)/3(v_abc_grid)
  filter inductance1/1(i_abc) -> [i_abc_filt]  "i_abc_filt"
  filter capacitance1/1(v_abc) -> [v_abc_filt]  "v_abc_filt"
  [Thetavsm] -> Inverse Park1/2(delta)
  Three-Phase V-I Measurement/1 -> [v_abc_grid]  "v_abc_grid"
  Inverse Park1/1(x_abc) -> Subsystem1/1(v_abc)
  Three-Phase V-I Measurement/2 -> [i_abc_grid]  "i_abc_grid"
  Gain5/1 -> Subsystem6/1(x_d+ix_q)
  Subsystem6/1(x_dq) -> Inverse Park1/1(x_dq)
  [vir] -> Gain5/1
  [Thetapll] -> Transformations (pu and dq)/6(Thetapll)
  [Thetavsm] -> Transformations (pu and dq)/5(Thetavsm)
  Transformations (pu and dq)/6(vo) -> Control System/6(vo)  "vo"
  Transformations (pu and dq)/5(vo_pll) -> Control System/5(vo_pll)  "vo_pll"
  Transformations (pu and dq)/4(q) -> Control System/4(q)  "q"
  Transformations (pu and dq)/3(p) -> Control System/3(p)  "p"
  Transformations (pu and dq)/1(io) -> Control System/1(io)  "io"
  Transformations (pu and dq)/2(il) -> Control System/2(il)  "il"
  Control System/1(thetapll) -> [Thetapll]
  Control System/3(vir) -> [vir]
  Control System/2(thetavsm) -> [Thetavsm]
  connections:
  Three-Phase Transformer (Two Windings)/LConn3 -- Three-Phase V-I Measurement/RConn3
  Three-Phase Transformer (Two Windings)/LConn2 -- Three-Phase V-I Measurement/RConn2
  Three-Phase Transformer (Two Windings)/LConn1 -- Three-Phase V-I Measurement/RConn1
  Three-Phase Transformer (Two Windings)/RConn3 -- c/RConn1
  Three-Phase Transformer (Two Windings)/RConn2 -- b/RConn1
  Three-Phase Transformer (Two Windings)/RConn1 -- a/RConn1
  Subsystem1/RConn3 -- filter inductance1/LConn3
  Subsystem1/RConn2 -- filter inductance1/LConn2
  Subsystem1/RConn1 -- filter inductance1/LConn1
  Three-Phase V-I Measurement/LConn2 -- filter capacitance1/LConn2 -- filter inductance1/RConn2
  Three-Phase V-I Measurement/LConn1 -- filter capacitance1/LConn1 -- filter inductance1/RConn1
  Three-Phase V-I Measurement/LConn3 -- filter capacitance1/LConn3 -- filter inductance1/RConn3

== system WF_offshore/WT_MF7 ==
  Control System : Subsystem  mask{Ts_control=cvtr.parameters.T_cont}
      mask prompts: Ts_control "Sample Time"
  Gain5 : Gain  Gain=cvtr.pu.Vb
  Inverse Park1 : Subsystem
  Subsystem1 : Subsystem
  Subsystem6 : Subsystem
  Three-Phase Transformer (Two Windings) : spsThreePhaseTransformerTwoWindingsLib/Three-Phase Transformer (Two Windings)  Winding1Connection=Yg  Winding2Connection=Yg  CoreType=Three single-phase transformers  SetSaturation=off  Hysteresis=off  DataFile='hysteresis'  SetInitialFlux=off  Measurements=None  UNITS=pu  NominalPower=[Sb_WT, f1 ]  Winding1=[ cvtr.parameters.Vnr ,r_tf_wt/2 , l_tf_wt/2]  Winding2=[ V_coll , r_tf_wt/2, l_tf_wt/2]  Rm=5000  Lm=0  L0=0.5  Saturation=[ 0,0 ; 0.0024,1.2 ; 1.0,1.52 ]  InitialFluxes=[ 0.8 , -0.8 , 0.7 ]  BreakLoop=off  DiscreteSolver=Trapezoidal iterative  DataType=off  TransfoNumber=1
  Three-Phase V-I Measurement : spsThreePhaseVIMeasurementLib/Three-Phase V-I Measurement  VoltageMeasurement=phase-to-ground  SetLabelV=off  LabelV=Vabc  Vpu=off  VpuLL=off  CurrentMeasurement=yes  SetLabelI=off  LabelI=Iabc  Ipu=off  Pbase=100e6  Vbase=500e3  OutputType=Complex  PhasorSimulation=off  PSBequivalent=0
  Transformations (pu and dq) : Subsystem
  filter capacitance1 : Subsystem
      settings: PortSchema="{\"entries\":[{\"content\":{\"sides\":[{\"content\":{\"connectorIds\":[\"LConn1\",\"LConn2\",\"LConn3\"]},\"type\":\"ConnectorPlacement.EquallySpacedRectSide\",\"uuid\":\"e81be3d5-6303-4565-8ca3-afc618f21d70\"},{\"content\":{\"connectorIds\":[],\"side\":\"RIGHT\"},\"type\":\"ConnectorPlacement.EquallySpacedRectSide\",\"uuid\":\"458d9030-e614-487d-87de-3e53be7c7da4\"},{\"content\":{\"connectorIds\":[],\"side\":\"TOP\"},\"type\":\"ConnectorPlacement.EquallySpacedRectSide\",\"uuid\":\"a29d66a0-f095-498d-bb9b-96c7f47699d3\"},{\"content\":{\"connectorIds\":[\"Out1\"],\"side\":\"BOTTOM\"},\"type\":\"ConnectorPlacement.EquallySpacedRectSide\",\"uuid\":\"afc68874-c098-43f5-9b37-53a3b484513b\"}]},\"type\":\"ConnectorPlacement.EquallySpacedConnector\",\"uuid\":\"37f495dd-1c12-4bb8-af72-7ef46bbd951c\"}],\"packageUris\":[\"http://schema.mathworks.com/mf0/Connector/R2020b\"],\"version\":\"1.0\"}"
  filter inductance1 : Subsystem
      settings: PortSchema="{\"entries\":[{\"content\":{\"sides\":[{\"content\":{\"connectorIds\":[\"LConn1\",\"LConn2\",\"LConn3\"]},\"type\":\"ConnectorPlacement.EquallySpacedRectSide\",\"uuid\":\"d3d60048-9578-4fa3-8d11-9c8a66a4b1f9\"},{\"content\":{\"connectorIds\":[\"RConn1\",\"RConn2\",\"RConn3\"],\"side\":\"RIGHT\"},\"type\":\"ConnectorPlacement.EquallySpacedRectSide\",\"uuid\":\"184a2c1d-36ab-46d1-99e4-db01aa31ec94\"},{\"content\":{\"connectorIds\":[\"Out1\"],\"side\":\"TOP\"},\"type\":\"ConnectorPlacement.EquallySpacedRectSide\",\"uuid\":\"db651021-9d7f-4124-8d21-ede853163467\"}]},\"type\":\"ConnectorPlacement.EquallySpacedConnector\",\"uuid\":\"723d0964-19fd-4dbe-91e3-e4ea0bb1cca9\"}],\"packageUris\":[\"http://schema.mathworks.com/mf0/Connector/R2020b\"],\"version\":\"1.0\"}"
  a : PMIOPort  Side=Right
  b : PMIOPort  Port=2  Side=Right
  c : PMIOPort  Port=3  Side=Right
  wires:
  Control System/2(thetavsm) -> [Thetavsm]
  Control System/3(vir) -> [vir]
  Control System/1(thetapll) -> [Thetapll]
  Transformations (pu and dq)/2(il) -> Control System/2(il)  "il"
  Transformations (pu and dq)/1(io) -> Control System/1(io)  "io"
  Transformations (pu and dq)/3(p) -> Control System/3(p)  "p"
  Transformations (pu and dq)/4(q) -> Control System/4(q)  "q"
  Transformations (pu and dq)/5(vo_pll) -> Control System/5(vo_pll)  "vo_pll"
  Transformations (pu and dq)/6(vo) -> Control System/6(vo)  "vo"
  [Thetavsm] -> Transformations (pu and dq)/5(Thetavsm)
  [Thetapll] -> Transformations (pu and dq)/6(Thetapll)
  [vir] -> Gain5/1
  Subsystem6/1(x_dq) -> Inverse Park1/1(x_dq)
  Gain5/1 -> Subsystem6/1(x_d+ix_q)
  Three-Phase V-I Measurement/2 -> [i_abc_grid]  "i_abc_grid"
  Inverse Park1/1(x_abc) -> Subsystem1/1(v_abc)
  Three-Phase V-I Measurement/1 -> [v_abc_grid]  "v_abc_grid"
  [Thetavsm] -> Inverse Park1/2(delta)
  filter capacitance1/1(v_abc) -> [v_abc_filt]  "v_abc_filt"
  filter inductance1/1(i_abc) -> [i_abc_filt]  "i_abc_filt"
  [v_abc_grid] -> Transformations (pu and dq)/3(v_abc_grid)
  [v_abc_filt] -> Transformations (pu and dq)/4(v_abc_filt)
  [i_abc_filt] -> Transformations (pu and dq)/2(i_abc_filt)
  [i_abc_grid] -> Transformations (pu and dq)/1(i_abc_grid)
  connections:
  filter inductance1/RConn3 -- filter capacitance1/LConn3 -- Three-Phase V-I Measurement/LConn3
  filter inductance1/RConn1 -- filter capacitance1/LConn1 -- Three-Phase V-I Measurement/LConn1
  filter inductance1/RConn2 -- filter capacitance1/LConn2 -- Three-Phase V-I Measurement/LConn2
  Subsystem1/RConn1 -- filter inductance1/LConn1
  Subsystem1/RConn2 -- filter inductance1/LConn2
  Subsystem1/RConn3 -- filter inductance1/LConn3
  Three-Phase Transformer (Two Windings)/RConn1 -- a/RConn1
  Three-Phase Transformer (Two Windings)/RConn2 -- b/RConn1
  Three-Phase Transformer (Two Windings)/RConn3 -- c/RConn1
  Three-Phase Transformer (Two Windings)/LConn1 -- Three-Phase V-I Measurement/RConn1
  Three-Phase Transformer (Two Windings)/LConn2 -- Three-Phase V-I Measurement/RConn2
  Three-Phase Transformer (Two Windings)/LConn3 -- Three-Phase V-I Measurement/RConn3

== system WF_offshore/WT_MF8 ==
  Control System : Subsystem  mask{Ts_control=cvtr.parameters.T_cont}
      mask prompts: Ts_control "Sample Time"
  Gain5 : Gain  Gain=cvtr.pu.Vb
  Inverse Park1 : Subsystem
  Subsystem1 : Subsystem
  Subsystem6 : Subsystem
  Three-Phase Transformer (Two Windings) : spsThreePhaseTransformerTwoWindingsLib/Three-Phase Transformer (Two Windings)  Winding1Connection=Yg  Winding2Connection=Yg  CoreType=Three single-phase transformers  SetSaturation=off  Hysteresis=off  DataFile='hysteresis'  SetInitialFlux=off  Measurements=None  UNITS=pu  NominalPower=[Sb_WT, f1 ]  Winding1=[ cvtr.parameters.Vnr ,r_tf_wt/2 , l_tf_wt/2]  Winding2=[ V_coll , r_tf_wt/2, l_tf_wt/2]  Rm=5000  Lm=0  L0=0.5  Saturation=[ 0,0 ; 0.0024,1.2 ; 1.0,1.52 ]  InitialFluxes=[ 0.8 , -0.8 , 0.7 ]  BreakLoop=off  DiscreteSolver=Trapezoidal iterative  DataType=off  TransfoNumber=1
  Three-Phase V-I Measurement : spsThreePhaseVIMeasurementLib/Three-Phase V-I Measurement  VoltageMeasurement=phase-to-ground  SetLabelV=off  LabelV=Vabc  Vpu=off  VpuLL=off  CurrentMeasurement=yes  SetLabelI=off  LabelI=Iabc  Ipu=off  Pbase=100e6  Vbase=500e3  OutputType=Complex  PhasorSimulation=off  PSBequivalent=0
  Transformations (pu and dq) : Subsystem
  filter capacitance1 : Subsystem
      settings: PortSchema="{\"entries\":[{\"content\":{\"sides\":[{\"content\":{\"connectorIds\":[\"LConn1\",\"LConn2\",\"LConn3\"]},\"type\":\"ConnectorPlacement.EquallySpacedRectSide\",\"uuid\":\"e81be3d5-6303-4565-8ca3-afc618f21d70\"},{\"content\":{\"connectorIds\":[],\"side\":\"RIGHT\"},\"type\":\"ConnectorPlacement.EquallySpacedRectSide\",\"uuid\":\"458d9030-e614-487d-87de-3e53be7c7da4\"},{\"content\":{\"connectorIds\":[],\"side\":\"TOP\"},\"type\":\"ConnectorPlacement.EquallySpacedRectSide\",\"uuid\":\"a29d66a0-f095-498d-bb9b-96c7f47699d3\"},{\"content\":{\"connectorIds\":[\"Out1\"],\"side\":\"BOTTOM\"},\"type\":\"ConnectorPlacement.EquallySpacedRectSide\",\"uuid\":\"afc68874-c098-43f5-9b37-53a3b484513b\"}]},\"type\":\"ConnectorPlacement.EquallySpacedConnector\",\"uuid\":\"37f495dd-1c12-4bb8-af72-7ef46bbd951c\"}],\"packageUris\":[\"http://schema.mathworks.com/mf0/Connector/R2020b\"],\"version\":\"1.0\"}"
  filter inductance1 : Subsystem
      settings: PortSchema="{\"entries\":[{\"content\":{\"sides\":[{\"content\":{\"connectorIds\":[\"LConn1\",\"LConn2\",\"LConn3\"]},\"type\":\"ConnectorPlacement.EquallySpacedRectSide\",\"uuid\":\"d3d60048-9578-4fa3-8d11-9c8a66a4b1f9\"},{\"content\":{\"connectorIds\":[\"RConn1\",\"RConn2\",\"RConn3\"],\"side\":\"RIGHT\"},\"type\":\"ConnectorPlacement.EquallySpacedRectSide\",\"uuid\":\"184a2c1d-36ab-46d1-99e4-db01aa31ec94\"},{\"content\":{\"connectorIds\":[\"Out1\"],\"side\":\"TOP\"},\"type\":\"ConnectorPlacement.EquallySpacedRectSide\",\"uuid\":\"db651021-9d7f-4124-8d21-ede853163467\"}]},\"type\":\"ConnectorPlacement.EquallySpacedConnector\",\"uuid\":\"723d0964-19fd-4dbe-91e3-e4ea0bb1cca9\"}],\"packageUris\":[\"http://schema.mathworks.com/mf0/Connector/R2020b\"],\"version\":\"1.0\"}"
  a : PMIOPort  Side=Right
  b : PMIOPort  Port=2  Side=Right
  c : PMIOPort  Port=3  Side=Right
  wires:
  [i_abc_grid] -> Transformations (pu and dq)/1(i_abc_grid)
  [i_abc_filt] -> Transformations (pu and dq)/2(i_abc_filt)
  [v_abc_filt] -> Transformations (pu and dq)/4(v_abc_filt)
  [v_abc_grid] -> Transformations (pu and dq)/3(v_abc_grid)
  filter inductance1/1(i_abc) -> [i_abc_filt]  "i_abc_filt"
  filter capacitance1/1(v_abc) -> [v_abc_filt]  "v_abc_filt"
  [Thetavsm] -> Inverse Park1/2(delta)
  Three-Phase V-I Measurement/1 -> [v_abc_grid]  "v_abc_grid"
  Inverse Park1/1(x_abc) -> Subsystem1/1(v_abc)
  Three-Phase V-I Measurement/2 -> [i_abc_grid]  "i_abc_grid"
  Gain5/1 -> Subsystem6/1(x_d+ix_q)
  Subsystem6/1(x_dq) -> Inverse Park1/1(x_dq)
  [vir] -> Gain5/1
  [Thetapll] -> Transformations (pu and dq)/6(Thetapll)
  [Thetavsm] -> Transformations (pu and dq)/5(Thetavsm)
  Transformations (pu and dq)/6(vo) -> Control System/6(vo)  "vo"
  Transformations (pu and dq)/5(vo_pll) -> Control System/5(vo_pll)  "vo_pll"
  Transformations (pu and dq)/4(q) -> Control System/4(q)  "q"
  Transformations (pu and dq)/3(p) -> Control System/3(p)  "p"
  Transformations (pu and dq)/1(io) -> Control System/1(io)  "io"
  Transformations (pu and dq)/2(il) -> Control System/2(il)  "il"
  Control System/1(thetapll) -> [Thetapll]
  Control System/3(vir) -> [vir]
  Control System/2(thetavsm) -> [Thetavsm]
  connections:
  Three-Phase Transformer (Two Windings)/LConn3 -- Three-Phase V-I Measurement/RConn3
  Three-Phase Transformer (Two Windings)/LConn2 -- Three-Phase V-I Measurement/RConn2
  Three-Phase Transformer (Two Windings)/LConn1 -- Three-Phase V-I Measurement/RConn1
  Three-Phase Transformer (Two Windings)/RConn3 -- c/RConn1
  Three-Phase Transformer (Two Windings)/RConn2 -- b/RConn1
  Three-Phase Transformer (Two Windings)/RConn1 -- a/RConn1
  Subsystem1/RConn3 -- filter inductance1/LConn3
  Subsystem1/RConn2 -- filter inductance1/LConn2
  Subsystem1/RConn1 -- filter inductance1/LConn1
  Three-Phase V-I Measurement/LConn2 -- filter capacitance1/LConn2 -- filter inductance1/RConn2
  Three-Phase V-I Measurement/LConn1 -- filter capacitance1/LConn1 -- filter inductance1/RConn1
  Three-Phase V-I Measurement/LConn3 -- filter capacitance1/LConn3 -- filter inductance1/RConn3
